simulink model "State_machine"  (R2017b)
settings: Solver=VariableStepAuto  StartTime=0.0  StopTime=10.0  RelTol=1e-3
settings Model: Creator=Kalana  LastModifiedBy=Kalana

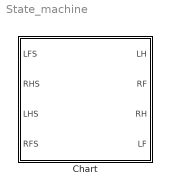
== system State_machine ==
  Chart : Stateflow chart  TreatAsAtomicUnit=on

== stateflow chart State_machine/Chart ==
  state LF_RH_swing
    entry: LF = 0
    RF = 1
    RH = 0
    LH = 1
  state Intermediate
    entry: LF = LF
    RF = RF
    RH = RH
    LH = LH
  state RF_LH_swing
    entry: LF = 1
    RF = 0
    RH = 1
    LH = 0
  LF_RH_swing -> Intermediate : [LFS + RHS]
  Intermediate -> RF_LH_swing [order 1] : [LFS*RHS]
  (default) -> LF_RH_swing
  Intermediate -> LF_RH_swing [order 2] : [RFS*LHS]
  RF_LH_swing -> Intermediate : [RFS+LHS]
  data: LH output; RF output; RH output; LF output; LFS input; RHS input; LHS input; RFS input
